simulink model "RBDmodel"  (R2023a)
settings: Solver=ode15s  StartTime=0.0  StopTime=4  FixedStep=0.0001  RelTol=1e-3  AbsTol=1e-3  EnableMultiTasking=on
model workspace (MAT data in the model file):
  C_Gimbal = 0.5
  C_IAP = 0.01
  IAP_Pa = 0
  K_Gimbal = 0
  K_IAP = 200
  LeftAbdominalMuscleForce = 0
  LeftBackMuscleForce = 0
  LeftTransverse1MuscleForce = 0
  LeftTransverse2MuscleForce = 0
  Moment_AR = 0
  Moment_FE = 7.5
  Moment_LB = 0
  RightAbdominalMuscleForce = 0
  RightBackMuscleForce = 0
  RightTransverse1MuscleForce = 0
  RightTransverse2MuscleForce = 0
  a = 1
  b = 1
  muscle_color = [0 0 1]
  muscle_radius = 1
libraries: checkpacklib x3, simulink x1
(part 1 of 2)
settings Model: PacingRate=0.110000  Creator=Siril TD  LastModifiedBy=siril
settings SolverCC: ZeroCrossAlgorithm=Adaptive  AutoInsertRateTranBlk=on
settings DataIOCC: LimitDataPoints=on  MaxDataPoints=50000  ReturnWorkspaceOutputsName=SDOSimTest_Log
settings OptimizationCC: LifeSpan=inf
settings DebuggingCC: IgnoredZcDiagnostic=none  UnconnectedInputMsg=warning  UnconnectedOutputMsg=warning  UnconnectedLineMsg=warning  AllowSymbolicDim=off  SFUnexpectedBacktrackingDiag=warning  SFNoUnconditionalDefaultTransitionDiag=warning  SFExecutionAtInitializationDiag=none  ArithmeticOperatorsInVariantConditions=warning
settings ModelReferenceCC: EnableRefExpFcnMdlSchedulingChecks=on
settings SFSimCC: SimUseLocalCustomCode=off  CustomCodeUndefinedFunction=UseInterfaceOnly
settings RTWCC: RTWUseLocalCustomCode=off  DLArmComputeVersion=19.05
settings CodeAppCC: StateflowObjectComments=on
settings GRTTargetCC: TargetLangStandard=C89/C90 (ANSI)
settings ConfigComp: CovMetricSettings=dw  CovSaveCumulativeToWorkspaceVar=on  CovSaveSingleToWorkspaceVar=on  CovExternalEMLEnable=off  CovSFcnEnable=off
settings SimscapeCC: SimscapeLogType=all  SimscapeLogSimulationStatistics=on  SimscapeLogDataHistory=10000

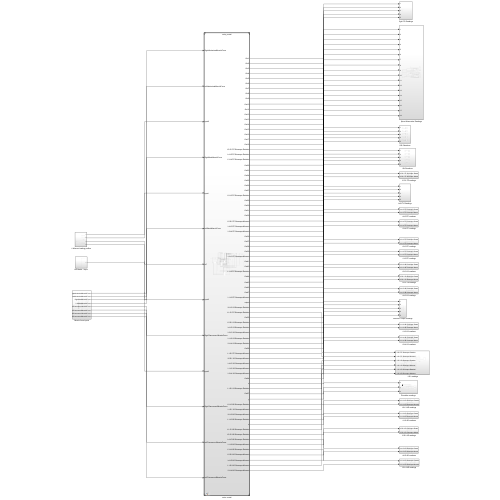
[thumbnail: Simulink's stored preview of the top-level diagram]
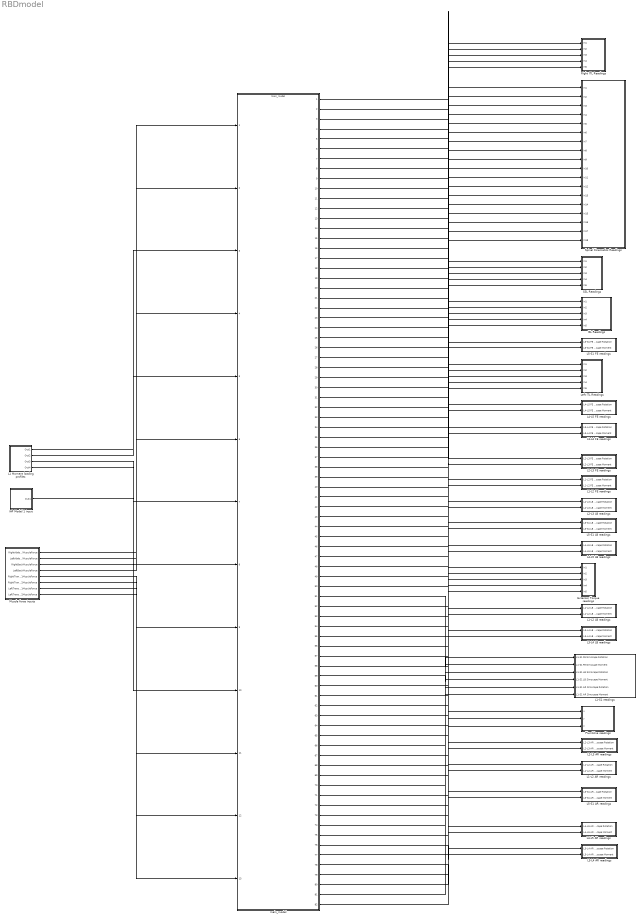
== system RBDmodel ==
  Extensor Torque readings : Subsystem
  IAP Model 1 input : Subsystem
  ISL Readings : Subsystem
  L1 Moment loading profiles : Subsystem
  L1-L2 AR readings : Subsystem
  L1-L2 FE readings : Subsystem
  L1-L2 LB readings : Subsystem
  L1-S1 readings : Subsystem
  L2-L3 AR readings : Subsystem
  L2-L3 FE readings : Subsystem
  L2-L3 LB readings : Subsystem
  L3-L4 AR readings : Subsystem
  L3-L4 FE readings : Subsystem
  L3-L4 LB readings : Subsystem
  L4-L5 AR readings : Subsystem
  L4-L5 FE readings : Subsystem
  L4-L5 LB readings : Subsystem
  L5-S1 AR readings : Subsystem
  L5-S1 FE readings : Subsystem
  L5-S1 LB readings : Subsystem
  Left ITL Readings : Subsystem
  Muscle force inputs : Subsystem
  Plumbline readings : Subsystem
  Right ITL Readings : Subsystem
  SSL Readings : Subsystem
  Spinal Kinematics Readings : Subsystem
  main_model : ModelReference  ModelNameDialog=main_model  SimulationMode=Normal  ModelReferenceVersion=6.155
  wires:
  main_model/20 -> L4-L5 FE readings/1(L4-L5 FE Simscape Rotation)
  main_model/67 -> Extensor Torque readings/5(In5)
  Muscle force inputs/4(LeftBackMuscleForce) -> main_model/6
  Muscle force inputs/3(RightBackMuscleForce) -> main_model/4
  L1 Moment loading profiles/1(Out1) -> main_model/3
  main_model/31 -> SSL Readings/4(In4)
  main_model/81 -> L1-S1 readings/6(L1-S1 AR Simscape Moment)
  main_model/56 -> L1-L2 LB readings/1(L1-L2 LB Simscape Rotation)
  L1 Moment loading profiles/2(Out2) -> main_model/5
  L1 Moment loading profiles/3(Out3) -> main_model/8
  main_model/50 -> L2-L3 LB readings/1(L2-L3 LB Simscape Rotation)
  main_model/6 -> SSL Readings/1(In1)
  L1 Moment loading profiles/4(Out4) -> main_model/10
  Muscle force inputs/1(RightAbdominalMuscleForce) -> main_model/1
  main_model/16 -> Left ITL Readings/2(In2)
  IAP Model 1 input/1(Out1) -> main_model/7
  Muscle force inputs/2(LeftAbdominalMuscleForce) -> main_model/2
  Muscle force inputs/5(RightTransverse1MuscleForce) -> main_model/9
  Muscle force inputs/6(RightTransverse2MuscleForce) -> main_model/11
  main_model/62 -> L1-L2 LB readings/2(L1-L2 LB Simscape Moment)
  Muscle force inputs/8(LeftTransverse2MuscleForce) -> main_model/13
  Muscle force inputs/7(LeftTransverse1MuscleForce) -> main_model/12
  main_model/63 -> L3-L4 LB readings/2(L3-L4 LB Simscape Moment)
  main_model/1 -> Spinal Kinematics Readings/1(In1)
  main_model/30 -> Spinal Kinematics Readings/13(In13)
  main_model/2 -> Spinal Kinematics Readings/2(In2)
  main_model/13 -> SSL Readings/2(In2)
  main_model/21 -> L3-L4 FE readings/1(L3-L4 FE Simscape Rotation)
  main_model/3 -> ISL Readings/1(In1)
  main_model/44 -> Spinal Kinematics Readings/17(In17)
  main_model/25 -> Spinal Kinematics Readings/11(In11)
  main_model/79 -> L5-S1 AR readings/2(L5-S1 AR Simscape Moment)
  main_model/4 -> Spinal Kinematics Readings/3(In3)
  main_model/5 -> Spinal Kinematics Readings/4(In4)
  main_model/77 -> L1-L2 AR readings/2(L1-L2 AR Simscape Moment)
  main_model/36 -> Spinal Kinematics Readings/14(In14)
  main_model/78 -> L3-L4 AR readings/1(L3-L4 AR Simscape Rotation)
  main_model/26 -> Left ITL Readings/3(In3)
  main_model/7 -> Spinal Kinematics Readings/5(In5)
  main_model/18 -> Right ITL Readings/3(In3)
  main_model/8 -> Left ITL Readings/1(In1)
  main_model/9 -> Right ITL Readings/1(In1)
  main_model/10 -> Spinal Kinematics Readings/6(In6)
  main_model/11 -> ISL Readings/2(In2)
  main_model/12 -> Spinal Kinematics Readings/7(In7)
  main_model/38 -> Left ITL Readings/4(In4)
  main_model/14 -> Right ITL Readings/2(In2)
  main_model/15 -> Spinal Kinematics Readings/8(In8)
  main_model/17 -> Spinal Kinematics Readings/9(In9)
  main_model/27 -> Right ITL Readings/4(In4)
  main_model/19 -> L5-S1 FE readings/1(L5-S1 FE Simscape Rotation)
  main_model/22 -> Spinal Kinematics Readings/10(In10)
  main_model/33 -> L5-S1 FE readings/2(L5-S1 FE Simscape Moment)
  main_model/23 -> ISL Readings/3(In3)
  main_model/45 -> Left ITL Readings/5(In5)
  main_model/24 -> SSL Readings/3(In3)
  main_model/28 -> L2-L3 FE readings/1(L2-L3 FE Simscape Rotation)
  main_model/29 -> Spinal Kinematics Readings/12(In12)
  main_model/32 -> Right ITL Readings/5(In5)
  main_model/34 -> L4-L5 FE readings/2(L4-L5 FE Simscape Moment)
  main_model/59 -> L1-S1 readings/2(L1-S1 FE Simscape Moment)
  main_model/35 -> L3-L4 FE readings/2(L3-L4 FE Simscape Moment)
  main_model/37 -> ISL Readings/4(In4)
  main_model/51 -> L1-S1 readings/1(L1-S1 FE Simscape Rotation)
  main_model/39 -> Spinal Kinematics Readings/15(In15)
  main_model/40 -> L2-L3 FE readings/2(L2-L3 FE Simscape Moment)
  main_model/41 -> Spinal Kinematics Readings/16(In16)
  main_model/42 -> SSL Readings/5(In5)
  main_model/43 -> L1-L2 FE readings/1(L1-L2 FE Simscape Rotation)
  main_model/46 -> Spinal Kinematics Readings/18(In18)
  main_model/47 -> ISL Readings/5(In5)
  main_model/48 -> L1-L2 FE readings/2(L1-L2 FE Simscape Moment)
  main_model/49 -> Extensor Torque readings/1(In1)
  main_model/52 -> Extensor Torque readings/2(In2)
  main_model/68 -> Plumbline readings/2(y)
  main_model/53 -> L5-S1 LB readings/1(L5-S1 LB Simscape Rotation)
  main_model/54 -> L4-L5 LB readings/1(L4-L5 LB Simscape Rotation)
  main_model/55 -> L2-L3 LB readings/2(L2-L3 LB Simscape Moment)
  main_model/57 -> L3-L4 LB readings/1(L3-L4 LB Simscape Rotation)
  main_model/58 -> Extensor Torque readings/3(In3)
  main_model/60 -> L5-S1 LB readings/2(L5-S1 LB Simscape Moment)
  main_model/61 -> L4-L5 LB readings/2(L4-L5 LB Simscape Moment)
  main_model/64 -> Extensor Torque readings/4(In4)
  main_model/65 -> Plumbline readings/1(x)
  main_model/66 -> L1-S1 readings/3(L1-S1 LB Simscape Rotation)
  main_model/69 -> L2-L3 AR readings/1(L2-L3 AR Simscape Rotation)
  main_model/70 -> L1-S1 readings/4(L1-S1 LB Simscape Moment)
  main_model/71 -> L2-L3 AR readings/2(L2-L3 AR Simscape Moment)
  main_model/72 -> L1-L2 AR readings/1(L1-L2 AR Simscape Rotation)
  main_model/73 -> Plumbline readings/3(z)
  main_model/74 -> L1-S1 readings/5(L1-S1 AR Simscape Rotation)
  main_model/75 -> L5-S1 AR readings/1(L5-S1 AR Simscape Rotation)
  main_model/76 -> L4-L5 AR readings/1(L4-L5 AR Simscape Rotation)
  main_model/80 -> L4-L5 AR readings/2(L4-L5 AR Simscape Moment)
  main_model/82 -> L3-L4 AR readings/2(L3-L4 AR Simscape Moment)

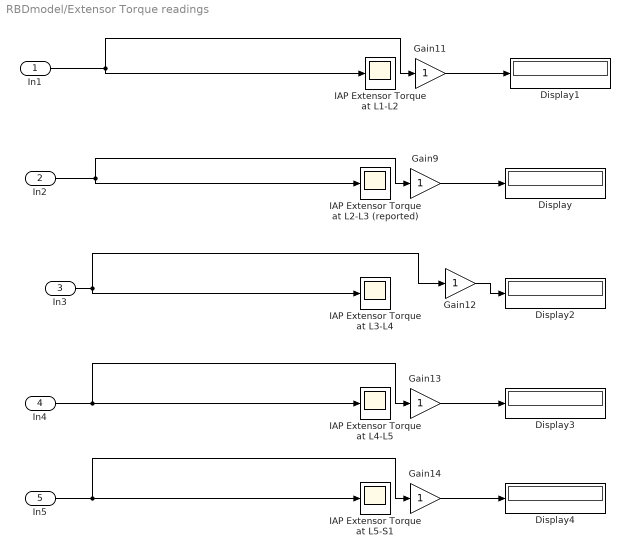
== system RBDmodel/Extensor Torque readings ==
  In1 : Inport
  In2 : Inport  Port=2
  In3 : Inport  Port=3
  In4 : Inport  Port=4
  In5 : Inport  Port=5
  Display{,1..4} (5 alike) : Display
      settings: Decimation=2
  Gain{9,11..14} (5 alike) : Gain
  IAP Extensor Torque at L1-L2 : Scope
  IAP Extensor Torque at L2-L3 (reported) : Scope
  IAP Extensor Torque at L3-L4 : Scope
  IAP Extensor Torque at L4-L5 : Scope
  IAP Extensor Torque at L5-S1 : Scope
  wires:
  Gain11/1 -> Display1/1
  Gain9/1 -> Display/1
  In5/1 -> Gain14/1, IAP Extensor Torque at L5-S1/1
  In2/1 -> Gain9/1, IAP Extensor Torque at L2-L3 (reported)/1
  Gain12/1 -> Display2/1
  In4/1 -> Gain13/1, IAP Extensor Torque at L4-L5/1
  In3/1 -> Gain12/1, IAP Extensor Torque at L3-L4/1
  Gain13/1 -> Display3/1
  In1/1 -> Gain11/1, IAP Extensor Torque at L1-L2/1
  Gain14/1 -> Display4/1

== system RBDmodel/IAP Model 1 input ==
  Constant96 : Constant  Value=IAP_Pa
  Out1 : Outport
  wires:
  Constant96/1 -> Out1/1

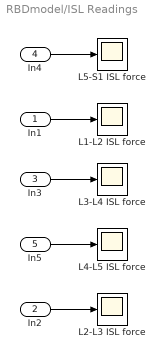
== system RBDmodel/ISL Readings ==
  In1 : Inport
  In2 : Inport  Port=2
  In3 : Inport  Port=3
  In4 : Inport  Port=4
  In5 : Inport  Port=5
  L1-L2 ISL force : Scope
  L2-L3 ISL force : Scope
  L3-L4 ISL force : Scope
  L4-L5 ISL force : Scope
  L5-S1 ISL force : Scope
  wires:
  In4/1 -> L5-S1 ISL force/1
  In2/1 -> L2-L3 ISL force/1
  In1/1 -> L1-L2 ISL force/1
  In3/1 -> L3-L4 ISL force/1
  In5/1 -> L4-L5 ISL force/1

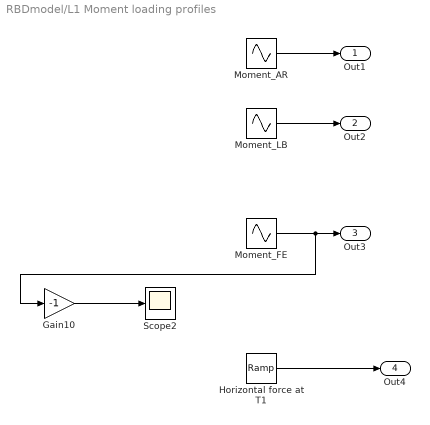
== system RBDmodel/L1 Moment loading profiles ==
  Gain10 : Gain  Gain=-1
  Horizontal force at T1 : simulink/Sources/Ramp  slope=0  start=0  InitialOutput=0
  Moment_AR : Sin  Amplitude=Moment_AR  SampleTime=0
  Moment_FE : Sin  Amplitude=-Moment_FE  SampleTime=0
  Moment_LB : Sin  Amplitude=-Moment_LB  SampleTime=0
  Scope2 : Scope
  Out1 : Outport
  Out2 : Outport  Port=2
  Out3 : Outport  Port=3
  Out4 : Outport  Port=4
  wires:
  Gain10/1 -> Scope2/1
  Horizontal force at T1/1 -> Out4/1
  Moment_LB/1 -> Out2/1
  Moment_AR/1 -> Out1/1
  Moment_FE/1 -> Gain10/1, Out3/1

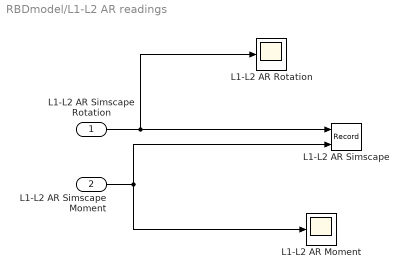
== system RBDmodel/L1-L2 AR readings ==
  L1-L2 AR Simscape Rotation : Inport
  L1-L2 AR Simscape Moment : Inport  Port=2
  L1-L2 AR Moment : Scope
  L1-L2 AR Rotation : Scope
  L1-L2 AR Simscape : Record  FileSettingsInternal="{\"entries\":[{\"content\":{\"excelSettings\":{\"content\":{},\"type\":\"Streamout.ExcelSettings\"}},\"type\":\"Streamout.FileSettingStorage\",\"uuid\":\"b28dc066-991e-4613-a00d-d29ff6d798a1\"}],\"packageUris\":[\"http://schema.mathworks.com/mf0/streamout_blocks/R2020a\"],\"version\":\"1.0\"}"  Layout=[1 1]  SignalsInternal="{\"entries\":[{\"content\":{\"signals\":[{\"content\":{\"blockPath\":[\"RBDmodel/L1-L2 AR readings/L1-L2 AR Simscape\"],\"dimensions\":[1],\"domain\":\"RBDmodel/L1-L2 AR readings/L1-L2 AR Simscape\",\"lineColor\":\"#ff6929\",\"port\":1,\"sid\":[\"\"],\"signalID\":1360,\"signalName\":\"L1-L2 AR Simscape Rotation\"},\"type\":\"RecordBlkView.Signal\",\"uuid\":\"012eb32e-fa43-42f2-9214-58300afc2241\"},{\"content\":{\"blockPath\":[\"RBDmodel/L1-L2 AR readings/L1-L2 AR Simscape\"],\"dimensions\":[1],\"domain\":\"RBDmodel/L1-L2 AR readings/L1-L2 AR Simscape\",\"lineColor\":\"#b746ff\",\"port\":2,\"sid\":[\"\"],\"signalID\":1364,\"signalName\":\"L1-L2 AR Simscape Moment\"},\"type\":\"RecordBlkView.Signal\",\"uuid\":\"1a3da7e1-f63f-4174-9c92-f6b8960343b7\"}]},\"type\":\"RecordBlkView.InputSignals\",\"uuid\":\"afe20b8d-c1d7-4091-a686-51fac02b3391\"}],\"packageUris\":[\"http://schema.mathworks.com/mf0/streamout_blocks/R2020a\"],\"version\":\"1.0\"}"  VisualizationBindings="{\"xyplotplugin\":{\"info\":[{\"series\":[],\"subplotID\":1}]}}"  CompatibilityTag=XY
  wires:
  L1-L2 AR Simscape Rotation/1 -> L1-L2 AR Simscape/1, L1-L2 AR Rotation/1
  L1-L2 AR Simscape Moment/1 -> L1-L2 AR Simscape/2, L1-L2 AR Moment/1

== system RBDmodel/L1-L2 FE readings ==
  L1-L2 FE Simscape Rotation : Inport
  L1-L2 FE Simscape Moment : Inport  Port=2
  L1-L2 FE Moment : Scope
  L1-L2 FE Rotation : Scope
  L1-L2 FE Simscape : Record  FileSettingsInternal="{\"entries\":[{\"content\":{\"excelSettings\":{\"content\":{},\"type\":\"Streamout.ExcelSettings\"}},\"type\":\"Streamout.FileSettingStorage\",\"uuid\":\"8ce7ea1e-727d-4085-a2f9-c3a4a6f5bb0a\"}],\"packageUris\":[\"http://schema.mathworks.com/mf0/streamout_blocks/R2020a\"],\"version\":\"1.0\"}"  Layout=[1 1]  SignalsInternal="{\"entries\":[{\"content\":{\"signals\":[{\"content\":{\"blockPath\":[\"RBDmodel/L1-L2 FE readings/L1-L2 FE Simscape\"],\"dimensions\":[1],\"domain\":\"RBDmodel/L1-L2 FE readings/L1-L2 FE Simscape\",\"lineColor\":\"#64d413\",\"port\":1,\"sid\":[\"\"],\"signalID\":1368,\"signalName\":\"L1-L2 FE Simscape Rotation\"},\"type\":\"RecordBlkView.Signal\",\"uuid\":\"14272d5e-dfd7-46c4-858f-28ca2b9ba15c\"},{\"content\":{\"blockPath\":[\"RBDmodel/L1-L2 FE readings/L1-L2 FE Simscape\"],\"dimensions\":[1],\"domain\":\"RBDmodel/L1-L2 FE readings/L1-L2 FE Simscape\",\"lineColor\":\"#ff13a6\",\"port\":2,\"sid\":[\"\"],\"signalID\":1372,\"signalName\":\"L1-L2 FE Simscape Moment\"},\"type\":\"RecordBlkView.Signal\",\"uuid\":\"e4bc809e-e80f-4428-925d-a05f0499dadb\"}]},\"type\":\"RecordBlkView.InputSignals\",\"uuid\":\"2abea1ec-8224-445c-bef5-2230a40efcc7\"}],\"packageUris\":[\"http://schema.mathworks.com/mf0/streamout_blocks/R2020a\"],\"version\":\"1.0\"}"  VisualizationBindings="{\"xyplotplugin\":{\"info\":[{\"series\":[],\"subplotID\":1}]}}"  CompatibilityTag=XY
  wires:
  L1-L2 FE Simscape Rotation/1 -> L1-L2 FE Simscape/1, L1-L2 FE Rotation/1
  L1-L2 FE Simscape Moment/1 -> L1-L2 FE Simscape/2, L1-L2 FE Moment/1

== system RBDmodel/L1-L2 LB readings ==
  L1-L2 LB Simscape Rotation : Inport
  L1-L2 LB Simscape Moment : Inport  Port=2
  L1-L2 LB Moment : Scope
  L1-L2 LB Rotation : Scope
  L1-L2 LB Simscape : Record  FileSettingsInternal="{\"entries\":[{\"content\":{\"excelSettings\":{\"content\":{},\"type\":\"Streamout.ExcelSettings\"}},\"type\":\"Streamout.FileSettingStorage\",\"uuid\":\"f91b6da8-1a5e-44a2-9c0b-2edd10b764e6\"}],\"packageUris\":[\"http://schema.mathworks.com/mf0/streamout_blocks/R2020a\"],\"version\":\"1.0\"}"  Layout=[1 1]  SignalsInternal="{\"entries\":[{\"content\":{\"signals\":[{\"content\":{\"blockPath\":[\"RBDmodel/L1-L2 LB readings/L1-L2 LB Simscape\"],\"dimensions\":[1],\"domain\":\"RBDmodel/L1-L2 LB readings/L1-L2 LB Simscape\",\"lineColor\":\"#fe330a\",\"port\":1,\"sid\":[\"\"],\"signalID\":1376,\"signalName\":\"L1-L2 LB Simscape Rotation\"},\"type\":\"RecordBlkView.Signal\",\"uuid\":\"621c9457-627a-42f5-82bc-3f73ddf07535\"},{\"content\":{\"blockPath\":[\"RBDmodel/L1-L2 LB readings/L1-L2 LB Simscape\"],\"dimensions\":[1],\"domain\":\"RBDmodel/L1-L2 LB readings/L1-L2 LB Simscape\",\"lineColor\":\"#22b573\",\"port\":2,\"sid\":[\"\"],\"signalID\":1380,\"signalName\":\"L1-L2 LB Simscape Moment\"},\"type\":\"RecordBlkView.Signal\",\"uuid\":\"2edc97f2-ad54-4451-8d37-6e34baaded79\"}]},\"type\":\"RecordBlkView.InputSignals\",\"uuid\":\"6599f76d-7cc0-48aa-b01b-dd0004c97a2e\"}],\"packageUris\":[\"http://schema.mathworks.com/mf0/streamout_blocks/R2020a\"],\"version\":\"1.0\"}"  VisualizationBindings="{\"xyplotplugin\":{\"info\":[{\"series\":[],\"subplotID\":1}]}}"  CompatibilityTag=XY
  wires:
  L1-L2 LB Simscape Moment/1 -> L1-L2 LB Simscape/2, L1-L2 LB Moment/1
  L1-L2 LB Simscape Rotation/1 -> L1-L2 LB Simscape/1, L1-L2 LB Rotation/1

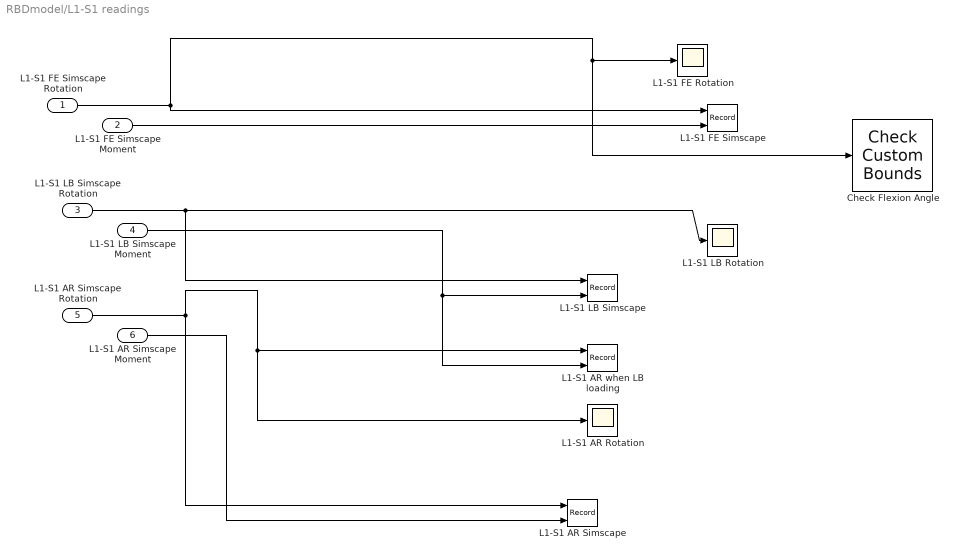
== system RBDmodel/L1-S1 readings ==
  L1-S1 FE Simscape Rotation : Inport
  L1-S1 FE Simscape Moment : Inport  Port=2
  L1-S1 LB Simscape Rotation : Inport  Port=3
  L1-S1 LB Simscape Moment : Inport  Port=4
  L1-S1 AR Simscape Rotation : Inport  Port=5
  L1-S1 AR Simscape Moment : Inport  Port=6
  Check Flexion Angle : checkpacklib/Check Custom Bounds  InstantiateOnLoad=on  enabled=off  stopWhenAssertionFail=off  export=off  ViewDlgPos=[100 200 510 390]  OpenViewOnLoad=off  LaunchViewOnOpen=off  TimeUnits=seconds  EnableUpperBound=on  UpperBoundTimes=[5 10]  UpperBoundAmplitudes=[51 51];  EnableLowerBound=on  LowerBoundTimes=[6 10]  LowerBoundAmplitudes=[49 49];
      settings: LibrarySourceBlock=sdolib/Signal Constraints/Check Custom Bounds
  L1-S1 AR Rotation : Scope
  L1-S1 AR Simscape : Record  FileSettingsInternal="{\"entries\":[{\"content\":{\"excelSettings\":{\"content\":{},\"type\":\"Streamout.ExcelSettings\"}},\"type\":\"Streamout.FileSettingStorage\",\"uuid\":\"b954e3b6-b992-4288-8e9e-83c0e0eed84f\"}],\"packageUris\":[\"http://schema.mathworks.com/mf0/streamout_blocks/R2020a\"],\"version\":\"1.0\"}"  Layout=[1 1]  SignalsInternal="{\"entries\":[{\"content\":{\"signals\":[{\"content\":{\"blockPath\":[\"RBDmodel/L1-S1 readings/L1-S1 AR Simscape\"],\"dimensions\":[1,1],\"domain\":\"RBDmodel/L1-S1 readings/L1-S1 AR Simscape\",\"lineColor\":\"#edb120\",\"port\":1,\"sid\":[\"\"],\"signalID\":1392,\"signalName\":\"L1-S1 AR Simscape Rotation\"},\"type\":\"RecordBlkView.Signal\",\"uuid\":\"797d9295-84dd-4e98-b2bd-abb01ffb65f1\"},{\"content\":{\"blockPath\":[\"RBDmodel/L1-S1 readings/L1-S1 AR Simscape\"],\"dimensions\":[1],\"domain\":\"RBDmodel/L1-S1 readings/L1-S1 AR Simscape\",\"lineColor\":\"#7e2f8e\",\"port\":2,\"sid\":[\"\"],\"signalID\":1396,\"signalName\":\"L1-S1 AR Simscape Moment\"},\"type\":\"RecordBlkView.Signal\",\"uuid\":\"1e31dda2-2ea6-4a38-a0e0-59a33a30f3aa\"}]},\"type\":\"RecordBlkView.InputSignals\",\"uuid\":\"77442a82-e315-402b-8b1a-300b9592f177\"}],\"packageUris\":[\"http://schema.mathworks.com/mf0/streamout_blocks/R2020a\"],\"version\":\"1.0\"}"  VisualizationBindings="{\"xyplotplugin\":{\"info\":[{\"series\":[],\"subplotID\":1}]}}"  CompatibilityTag=XY
  L1-S1 AR when LB loading : Record  FileSettingsInternal="{\"entries\":[{\"content\":{\"excelSettings\":{\"content\":{},\"type\":\"Streamout.ExcelSettings\"}},\"type\":\"Streamout.FileSettingStorage\",\"uuid\":\"7c9a55b9-26e2-4dee-8ab6-75e3d662341a\"}],\"packageUris\":[\"http://schema.mathworks.com/mf0/streamout_blocks/R2020a\"],\"version\":\"1.0\"}"  Layout=[1 1]  SignalsInternal="{\"entries\":[{\"content\":{\"signals\":[{\"content\":{\"blockPath\":[\"RBDmodel/L1-S1 readings/L1-S1 AR when LB loading\"],\"dimensions\":[1,1],\"domain\":\"RBDmodel/L1-S1 readings/L1-S1 AR when LB loading\",\"lineColor\":\"#77ac30\",\"port\":1,\"sid\":[\"\"],\"signalID\":1400,\"signalName\":\"L1-S1 AR Simscape Rotation\"},\"type\":\"RecordBlkView.Signal\",\"uuid\":\"fc9ea2b7-01a5-4fec-8c12-8ed0258352bf\"},{\"content\":{\"blockPath\":[\"RBDmodel/L1-S1 readings/L1-S1 AR when LB loading\"],\"dimensions\":[1],\"domain\":\"RBDmodel/L1-S1 readings/L1-S1 AR when LB loading\",\"lineColor\":\"#4dbeee\",\"port\":2,\"sid\":[\"\"],\"signalID\":1404,\"signalName\":\"L1-S1 LB Simscape Moment\"},\"type\":\"RecordBlkView.Signal\",\"uuid\":\"99554ea6-9241-406f-a7ff-00c072a0b4e4\"}]},\"type\":\"RecordBlkView.InputSignals\",\"uuid\":\"3f4efdd9-c46f-425d-a98a-f481f6a35fee\"}],\"packageUris\":[\"http://schema.mathworks.com/mf0/streamout_blocks/R2020a\"],\"version\":\"1.0\"}"  VisualizationBindings="{\"xyplotplugin\":{\"info\":[{\"series\":[],\"subplotID\":1}]}}"  CompatibilityTag=XY
  L1-S1 FE Rotation : Scope
  L1-S1 FE Simscape : Record  FileSettingsInternal="{\"entries\":[{\"content\":{\"excelSettings\":{\"content\":{},\"type\":\"Streamout.ExcelSettings\"}},\"type\":\"Streamout.FileSettingStorage\",\"uuid\":\"4277ec63-d6bc-434d-a603-e60f5b770cfc\"}],\"packageUris\":[\"http://schema.mathworks.com/mf0/streamout_blocks/R2020a\"],\"version\":\"1.0\"}"  Layout=[1 1]  SignalsInternal="{\"entries\":[{\"content\":{\"signals\":[{\"content\":{\"blockPath\":[\"RBDmodel/L1-S1 readings/L1-S1 FE Simscape\"],\"dimensions\":[1,1],\"domain\":\"RBDmodel/L1-S1 readings/L1-S1 FE Simscape\",\"lineColor\":\"#0072bd\",\"port\":1,\"sid\":[\"\"],\"signalID\":1384,\"signalName\":\"L1-S1 FE Simscape Rotation\"},\"type\":\"RecordBlkView.Signal\",\"uuid\":\"b05b0e40-1441-4de0-b556-a25aa3c4cf09\"},{\"content\":{\"blockPath\":[\"RBDmodel/L1-S1 readings/L1-S1 FE Simscape\"],\"dimensions\":[1],\"domain\":\"RBDmodel/L1-S1 readings/L1-S1 FE Simscape\",\"lineColor\":\"#d95319\",\"port\":2,\"sid\":[\"\"],\"signalID\":1388,\"signalName\":\"L1-S1 FE Simscape Moment\"},\"type\":\"RecordBlkView.Signal\",\"uuid\":\"32cda3f8-6cbe-4181-ae22-8066d64c7fad\"}]},\"type\":\"RecordBlkView.InputSignals\",\"uuid\":\"42077291-aac0-4e4f-98f6-8f120505d114\"}],\"packageUris\":[\"http://schema.mathworks.com/mf0/streamout_blocks/R2020a\"],\"version\":\"1.0\"}"  VisualizationBindings="{\"xyplotplugin\":{\"info\":[{\"series\":[],\"subplotID\":1}]}}"  CompatibilityTag=XY
  L1-S1 LB Rotation : Scope
  L1-S1 LB Simscape : Record  FileSettingsInternal="{\"entries\":[{\"content\":{\"excelSettings\":{\"content\":{},\"type\":\"Streamout.ExcelSettings\"}},\"type\":\"Streamout.FileSettingStorage\",\"uuid\":\"d051a5cc-fb2e-466c-bd05-561f4ba50a96\"}],\"packageUris\":[\"http://schema.mathworks.com/mf0/streamout_blocks/R2020a\"],\"version\":\"1.0\"}"  Layout=[1 1]  SignalsInternal="{\"entries\":[{\"content\":{\"signals\":[{\"content\":{\"blockPath\":[\"RBDmodel/L1-S1 readings/L1-S1 LB Simscape\"],\"dimensions\":[1,1],\"domain\":\"RBDmodel/L1-S1 readings/L1-S1 LB Simscape\",\"lineColor\":\"#a2142f\",\"port\":1,\"sid\":[\"\"],\"signalID\":1408,\"signalName\":\"L1-S1 LB Simscape Rotation\"},\"type\":\"RecordBlkView.Signal\",\"uuid\":\"a043fbb2-f081-461b-bfbf-22b79d9b12f8\"},{\"content\":{\"blockPath\":[\"RBDmodel/L1-S1 readings/L1-S1 LB Simscape\"],\"dimensions\":[1],\"domain\":\"RBDmodel/L1-S1 readings/L1-S1 LB Simscape\",\"lineColor\":\"#139fff\",\"port\":2,\"sid\":[\"\"],\"signalID\":1412,\"signalName\":\"L1-S1 LB Simscape Moment\"},\"type\":\"RecordBlkView.Signal\",\"uuid\":\"92bbd904-5685-4112-b61d-6e93200ea034\"}]},\"type\":\"RecordBlkView.InputSignals\",\"uuid\":\"6b8d1cb8-5b8d-4fed-9469-309b6002e987\"}],\"packageUris\":[\"http://schema.mathworks.com/mf0/streamout_blocks/R2020a\"],\"version\":\"1.0\"}"  VisualizationBindings="{\"xyplotplugin\":{\"info\":[{\"series\":[],\"subplotID\":1}]}}"  CompatibilityTag=XY
  wires:
  L1-S1 LB Simscape Rotation/1 -> L1-S1 LB Simscape/1, L1-S1 LB Rotation/1
  L1-S1 FE Simscape Rotation/1 -> Check Flexion Angle/1, L1-S1 FE Rotation/1, L1-S1 FE Simscape/1
  L1-S1 AR Simscape Rotation/1 -> L1-S1 AR when LB loading/1, L1-S1 AR Rotation/1, L1-S1 AR Simscape/1
  L1-S1 LB Simscape Moment/1 -> L1-S1 LB Simscape/2, L1-S1 AR when LB loading/2
  L1-S1 FE Simscape Moment/1 -> L1-S1 FE Simscape/2
  L1-S1 AR Simscape Moment/1 -> L1-S1 AR Simscape/2

== system RBDmodel/L2-L3 AR readings ==
  L2-L3 AR Simscape Rotation : Inport
  L2-L3 AR Simscape Moment : Inport  Port=2
  L2-L3 AR Moment : Scope
  L2-L3 AR Rotation : Scope
  L2-L3 AR Simscape : Record  FileSettingsInternal="{\"entries\":[{\"content\":{\"excelSettings\":{\"content\":{},\"type\":\"Streamout.ExcelSettings\"}},\"type\":\"Streamout.FileSettingStorage\",\"uuid\":\"1b3dca45-e25d-4c43-83f1-4bff6aa87f96\"}],\"packageUris\":[\"http://schema.mathworks.com/mf0/streamout_blocks/R2020a\"],\"version\":\"1.0\"}"  Layout=[1 1]  SignalsInternal="{\"entries\":[{\"content\":{\"signals\":[{\"content\":{\"blockPath\":[\"RBDmodel/L2-L3 AR readings/L2-L3 AR Simscape\"],\"dimensions\":[1],\"domain\":\"RBDmodel/L2-L3 AR readings/L2-L3 AR Simscape\",\"lineColor\":\"#ff6929\",\"port\":1,\"sid\":[\"\"],\"signalID\":1416,\"signalName\":\"L2-L3 AR Simscape Rotation\"},\"type\":\"RecordBlkView.Signal\",\"uuid\":\"e70d2628-5331-497c-85aa-337cd48ba713\"},{\"content\":{\"blockPath\":[\"RBDmodel/L2-L3 AR readings/L2-L3 AR Simscape\"],\"dimensions\":[1],\"domain\":\"RBDmodel/L2-L3 AR readings/L2-L3 AR Simscape\",\"lineColor\":\"#b746ff\",\"port\":2,\"sid\":[\"\"],\"signalID\":1420,\"signalName\":\"L2-L3 AR Simscape Moment\"},\"type\":\"RecordBlkView.Signal\",\"uuid\":\"af39c3ea-201a-40c1-a483-dfe03c7ab99b\"}]},\"type\":\"RecordBlkView.InputSignals\",\"uuid\":\"a20d0424-911b-47f8-ba88-4e87d1c9c6ef\"}],\"packageUris\":[\"http://schema.mathworks.com/mf0/streamout_blocks/R2020a\"],\"version\":\"1.0\"}"  VisualizationBindings="{\"xyplotplugin\":{\"info\":[{\"series\":[],\"subplotID\":1}]}}"  CompatibilityTag=XY
  wires:
  L2-L3 AR Simscape Rotation/1 -> L2-L3 AR Simscape/1, L2-L3 AR Rotation/1
  L2-L3 AR Simscape Moment/1 -> L2-L3 AR Simscape/2, L2-L3 AR Moment/1

== system RBDmodel/L2-L3 FE readings ==
  L2-L3 FE Simscape Rotation : Inport
  L2-L3 FE Simscape Moment : Inport  Port=2
  L2-L3 FE Moment : Scope
  L2-L3 FE Rotation : Scope
  L2-L3 FE Simscape : Record  FileSettingsInternal="{\"entries\":[{\"content\":{\"excelSettings\":{\"content\":{},\"type\":\"Streamout.ExcelSettings\"}},\"type\":\"Streamout.FileSettingStorage\",\"uuid\":\"a8dbeb5b-ff1f-49c5-807a-ed83070a13e0\"}],\"packageUris\":[\"http://schema.mathworks.com/mf0/streamout_blocks/R2020a\"],\"version\":\"1.0\"}"  Layout=[1 1]  SignalsInternal="{\"entries\":[{\"content\":{\"signals\":[{\"content\":{\"blockPath\":[\"RBDmodel/L2-L3 FE readings/L2-L3 FE Simscape\"],\"dimensions\":[1],\"domain\":\"RBDmodel/L2-L3 FE readings/L2-L3 FE Simscape\",\"lineColor\":\"#64d413\",\"port\":1,\"sid\":[\"\"],\"signalID\":1424,\"signalName\":\"L2-L3 FE Simscape Rotation\"},\"type\":\"RecordBlkView.Signal\",\"uuid\":\"610a7a81-37ad-4730-b63c-a5761efec7a8\"},{\"content\":{\"blockPath\":[\"RBDmodel/L2-L3 FE readings/L2-L3 FE Simscape\"],\"dimensions\":[1],\"domain\":\"RBDmodel/L2-L3 FE readings/L2-L3 FE Simscape\",\"lineColor\":\"#ff13a6\",\"port\":2,\"sid\":[\"\"],\"signalID\":1428,\"signalName\":\"L2-L3 FE Simscape Moment\"},\"type\":\"RecordBlkView.Signal\",\"uuid\":\"85b15c0e-062c-4388-a88e-8c4ab91d18f2\"}]},\"type\":\"RecordBlkView.InputSignals\",\"uuid\":\"8aa61301-8cd2-4db8-affe-7794c216c0d9\"}],\"packageUris\":[\"http://schema.mathworks.com/mf0/streamout_blocks/R2020a\"],\"version\":\"1.0\"}"  VisualizationBindings="{\"xyplotplugin\":{\"info\":[{\"series\":[],\"subplotID\":1}]}}"  CompatibilityTag=XY
  wires:
  L2-L3 FE Simscape Rotation/1 -> L2-L3 FE Simscape/1, L2-L3 FE Rotation/1
  L2-L3 FE Simscape Moment/1 -> L2-L3 FE Simscape/2, L2-L3 FE Moment/1

== system RBDmodel/L2-L3 LB readings ==
  L2-L3 LB Simscape Rotation : Inport
  L2-L3 LB Simscape Moment : Inport  Port=2
  L2-L3 LB Moment : Scope
  L2-L3 LB Rotation : Scope
  L2-L3 LB Simscape : Record  FileSettingsInternal="{\"entries\":[{\"content\":{\"excelSettings\":{\"content\":{},\"type\":\"Streamout.ExcelSettings\"}},\"type\":\"Streamout.FileSettingStorage\",\"uuid\":\"ebb8c812-f4e5-4f1b-bb26-5cc9383d42b0\"}],\"packageUris\":[\"http://schema.mathworks.com/mf0/streamout_blocks/R2020a\"],\"version\":\"1.0\"}"  Layout=[1 1]  SignalsInternal="{\"entries\":[{\"content\":{\"signals\":[{\"content\":{\"blockPath\":[\"RBDmodel/L2-L3 LB readings/L2-L3 LB Simscape\"],\"dimensions\":[1],\"domain\":\"RBDmodel/L2-L3 LB readings/L2-L3 LB Simscape\",\"lineColor\":\"#fe330a\",\"port\":1,\"sid\":[\"\"],\"signalID\":1432,\"signalName\":\"L2-L3 LB Simscape Rotation\"},\"type\":\"RecordBlkView.Signal\",\"uuid\":\"54576e5c-c28b-43e4-9224-e94e1705c380\"},{\"content\":{\"blockPath\":[\"RBDmodel/L2-L3 LB readings/L2-L3 LB Simscape\"],\"dimensions\":[1],\"domain\":\"RBDmodel/L2-L3 LB readings/L2-L3 LB Simscape\",\"lineColor\":\"#22b573\",\"port\":2,\"sid\":[\"\"],\"signalID\":1436,\"signalName\":\"L2-L3 LB Simscape Moment\"},\"type\":\"RecordBlkView.Signal\",\"uuid\":\"a9740b53-4785-48f0-9501-c2b6069bd585\"}]},\"type\":\"RecordBlkView.InputSignals\",\"uuid\":\"1bea8120-5db7-433b-aae0-c9997d8e4541\"}],\"packageUris\":[\"http://schema.mathworks.com/mf0/streamout_blocks/R2020a\"],\"version\":\"1.0\"}"  VisualizationBindings="{\"xyplotplugin\":{\"info\":[{\"series\":[],\"subplotID\":1}]}}"  CompatibilityTag=XY
  wires:
  L2-L3 LB Simscape Rotation/1 -> L2-L3 LB Simscape/1, L2-L3 LB Rotation/1
  L2-L3 LB Simscape Moment/1 -> L2-L3 LB Simscape/2, L2-L3 LB Moment/1

== system RBDmodel/L3-L4 AR readings ==
  L3-L4 AR Simscape Rotation : Inport
  L3-L4 AR Simscape Moment : Inport  Port=2
  L3-L4 AR Moment : Scope
  L3-L4 AR Rotation : Scope
  L3-L4 AR Simscape : Record  FileSettingsInternal="{\"entries\":[{\"content\":{\"excelSettings\":{\"content\":{},\"type\":\"Streamout.ExcelSettings\"}},\"type\":\"Streamout.FileSettingStorage\",\"uuid\":\"0d852f55-8e65-459e-b217-a04e03d20f27\"}],\"packageUris\":[\"http://schema.mathworks.com/mf0/streamout_blocks/R2020a\"],\"version\":\"1.0\"}"  Layout=[1 1]  SignalsInternal="{\"entries\":[{\"content\":{\"signals\":[{\"content\":{\"blockPath\":[\"RBDmodel/L3-L4 AR readings/L3-L4 AR Simscape\"],\"dimensions\":[1],\"domain\":\"RBDmodel/L3-L4 AR readings/L3-L4 AR Simscape\",\"lineColor\":\"#0072bd\",\"port\":1,\"sid\":[\"\"],\"signalID\":1440,\"signalName\":\"L3-L4 AR Simscape Rotation\"},\"type\":\"RecordBlkView.Signal\",\"uuid\":\"751fb338-a416-415f-9a67-fed1a750ab96\"},{\"content\":{\"blockPath\":[\"RBDmodel/L3-L4 AR readings/L3-L4 AR Simscape\"],\"dimensions\":[1],\"domain\":\"RBDmodel/L3-L4 AR readings/L3-L4 AR Simscape\",\"lineColor\":\"#d95319\",\"port\":2,\"sid\":[\"\"],\"signalID\":1444,\"signalName\":\"L3-L4 AR Simscape Moment\"},\"type\":\"RecordBlkView.Signal\",\"uuid\":\"1623f842-dbcd-465f-acad-6502715e33f9\"}]},\"type\":\"RecordBlkView.InputSignals\",\"uuid\":\"4d0e25ad-78aa-47cf-9e32-c99cd5c12085\"}],\"packageUris\":[\"http://schema.mathworks.com/mf0/streamout_blocks/R2020a\"],\"version\":\"1.0\"}"  VisualizationBindings="{\"xyplotplugin\":{\"info\":[{\"series\":[],\"subplotID\":1}]}}"  CompatibilityTag=XY
  wires:
  L3-L4 AR Simscape Rotation/1 -> L3-L4 AR Simscape/1, L3-L4 AR Rotation/1
  L3-L4 AR Simscape Moment/1 -> L3-L4 AR Simscape/2, L3-L4 AR Moment/1

== system RBDmodel/L3-L4 FE readings ==
  L3-L4 FE Simscape Rotation : Inport
  L3-L4 FE Simscape Moment : Inport  Port=2
  L3-L4 FE Moment : Scope
  L3-L4 FE Rotation : Scope
  L3-L4 FE Simscape : Record  FileSettingsInternal="{\"entries\":[{\"content\":{\"excelSettings\":{\"content\":{},\"type\":\"Streamout.ExcelSettings\"}},\"type\":\"Streamout.FileSettingStorage\",\"uuid\":\"4a97007c-b2c5-4a2b-a22c-db91ba4f89a2\"}],\"packageUris\":[\"http://schema.mathworks.com/mf0/streamout_blocks/R2020a\"],\"version\":\"1.0\"}"  Layout=[1 1]  SignalsInternal="{\"entries\":[{\"content\":{\"signals\":[{\"content\":{\"blockPath\":[\"RBDmodel/L3-L4 FE readings/L3-L4 FE Simscape\"],\"dimensions\":[1],\"domain\":\"RBDmodel/L3-L4 FE readings/L3-L4 FE Simscape\",\"lineColor\":\"#edb120\",\"port\":1,\"sid\":[\"\"],\"signalID\":1448,\"signalName\":\"L3-L4 FE Simscape Rotation\"},\"type\":\"RecordBlkView.Signal\",\"uuid\":\"77a480f7-8074-47be-8fdf-a8caa3efc9ea\"},{\"content\":{\"blockPath\":[\"RBDmodel/L3-L4 FE readings/L3-L4 FE Simscape\"],\"dimensions\":[1],\"domain\":\"RBDmodel/L3-L4 FE readings/L3-L4 FE Simscape\",\"lineColor\":\"#7e2f8e\",\"port\":2,\"sid\":[\"\"],\"signalID\":1452,\"signalName\":\"L3-L4 FE Simscape Moment\"},\"type\":\"RecordBlkView.Signal\",\"uuid\":\"bbaedb1d-6b55-4b73-9374-f86fb5d1519f\"}]},\"type\":\"RecordBlkView.InputSignals\",\"uuid\":\"8922dd5c-60c6-4104-bd66-638812c4d691\"}],\"packageUris\":[\"http://schema.mathworks.com/mf0/streamout_blocks/R2020a\"],\"version\":\"1.0\"}"  VisualizationBindings="{\"xyplotplugin\":{\"info\":[{\"series\":[],\"subplotID\":1}]}}"  CompatibilityTag=XY
  wires:
  L3-L4 FE Simscape Rotation/1 -> L3-L4 FE Simscape/1, L3-L4 FE Rotation/1
  L3-L4 FE Simscape Moment/1 -> L3-L4 FE Simscape/2, L3-L4 FE Moment/1

== system RBDmodel/L3-L4 LB readings ==
  L3-L4 LB Simscape Rotation : Inport
  L3-L4 LB Simscape Moment : Inport  Port=2
  L3-L4 LB Moment : Scope
  L3-L4 LB Rotation : Scope
  L3-L4 LB Simscape : Record  FileSettingsInternal="{\"entries\":[{\"content\":{\"excelSettings\":{\"content\":{},\"type\":\"Streamout.ExcelSettings\"}},\"type\":\"Streamout.FileSettingStorage\",\"uuid\":\"1c058524-eb60-4b6f-8fef-1b5d5278ec82\"}],\"packageUris\":[\"http://schema.mathworks.com/mf0/streamout_blocks/R2020a\"],\"version\":\"1.0\"}"  Layout=[1 1]  SignalsInternal="{\"entries\":[{\"content\":{\"signals\":[{\"content\":{\"blockPath\":[\"RBDmodel/L3-L4 LB readings/L3-L4 LB Simscape\"],\"dimensions\":[1],\"domain\":\"RBDmodel/L3-L4 LB readings/L3-L4 LB Simscape\",\"lineColor\":\"#77ac30\",\"port\":1,\"sid\":[\"\"],\"signalID\":1456,\"signalName\":\"L3-L4 LB Simscape Rotation\"},\"type\":\"RecordBlkView.Signal\",\"uuid\":\"2dc6856a-0e52-4543-b3ac-6e8ed32a5d94\"},{\"content\":{\"blockPath\":[\"RBDmodel/L3-L4 LB readings/L3-L4 LB Simscape\"],\"dimensions\":[1],\"domain\":\"RBDmodel/L3-L4 LB readings/L3-L4 LB Simscape\",\"lineColor\":\"#4dbeee\",\"port\":2,\"sid\":[\"\"],\"signalID\":1460,\"signalName\":\"L3-L4 LB Simscape Moment\"},\"type\":\"RecordBlkView.Signal\",\"uuid\":\"eb138c01-ee40-4649-b1c0-29d03f62432c\"}]},\"type\":\"RecordBlkView.InputSignals\",\"uuid\":\"c7c7ce33-7e8f-4fb1-9a81-42256479e298\"}],\"packageUris\":[\"http://schema.mathworks.com/mf0/streamout_blocks/R2020a\"],\"version\":\"1.0\"}"  VisualizationBindings="{\"xyplotplugin\":{\"info\":[{\"series\":[],\"subplotID\":1}]}}"  CompatibilityTag=XY
  wires:
  L3-L4 LB Simscape Rotation/1 -> L3-L4 LB Simscape/1, L3-L4 LB Rotation/1
  L3-L4 LB Simscape Moment/1 -> L3-L4 LB Simscape/2, L3-L4 LB Moment/1

== system RBDmodel/L4-L5 AR readings ==
  L4-L5 AR Simscape Rotation : Inport
  L4-L5 AR Simscape Moment : Inport  Port=2
  L4-L5 AR Moment : Scope
  L4-L5 AR Rotation : Scope
  L4-L5 AR Simscape : Record  FileSettingsInternal="{\"entries\":[{\"content\":{\"excelSettings\":{\"content\":{},\"type\":\"Streamout.ExcelSettings\"}},\"type\":\"Streamout.FileSettingStorage\",\"uuid\":\"22ee5429-b0dc-4563-83b8-15fc97b18f1f\"}],\"packageUris\":[\"http://schema.mathworks.com/mf0/streamout_blocks/R2020a\"],\"version\":\"1.0\"}"  Layout=[1 1]  SignalsInternal="{\"entries\":[{\"content\":{\"signals\":[{\"content\":{\"blockPath\":[\"RBDmodel/L4-L5 AR readings/L4-L5 AR Simscape\"],\"dimensions\":[1],\"domain\":\"RBDmodel/L4-L5 AR readings/L4-L5 AR Simscape\",\"lineColor\":\"#a2142f\",\"port\":1,\"sid\":[\"\"],\"signalID\":1464,\"signalName\":\"L4-L5 AR Simscape Rotation\"},\"type\":\"RecordBlkView.Signal\",\"uuid\":\"878d9bd7-08b6-4dbd-bbe6-ed022d721c95\"},{\"content\":{\"blockPath\":[\"RBDmodel/L4-L5 AR readings/L4-L5 AR Simscape\"],\"dimensions\":[1],\"domain\":\"RBDmodel/L4-L5 AR readings/L4-L5 AR Simscape\",\"lineColor\":\"#139fff\",\"port\":2,\"sid\":[\"\"],\"signalID\":1468,\"signalName\":\"L4-L5 AR Simscape Moment\"},\"type\":\"RecordBlkView.Signal\",\"uuid\":\"8a0298d5-c88a-476b-907c-fa990a76708f\"}]},\"type\":\"RecordBlkView.InputSignals\",\"uuid\":\"d6c75fef-9b3d-4599-8e28-137f3ee6693b\"}],\"packageUris\":[\"http://schema.mathworks.com/mf0/streamout_blocks/R2020a\"],\"version\":\"1.0\"}"  VisualizationBindings="{\"xyplotplugin\":{\"info\":[{\"series\":[],\"subplotID\":1}]}}"  CompatibilityTag=XY
  wires:
  L4-L5 AR Simscape Moment/1 -> L4-L5 AR Simscape/2, L4-L5 AR Moment/1
  L4-L5 AR Simscape Rotation/1 -> L4-L5 AR Simscape/1, L4-L5 AR Rotation/1

== system RBDmodel/L4-L5 FE readings ==
  L4-L5 FE Simscape Rotation : Inport
  L4-L5 FE Simscape Moment : Inport  Port=2
  L4-L5 FE Moment : Scope
  L4-L5 FE Rotation : Scope
  L4-L5 FE Simscape : Record  FileSettingsInternal="{\"entries\":[{\"content\":{\"excelSettings\":{\"content\":{},\"type\":\"Streamout.ExcelSettings\"}},\"type\":\"Streamout.FileSettingStorage\",\"uuid\":\"f454a2f2-99ca-4f18-a30c-f3205bc0580a\"}],\"packageUris\":[\"http://schema.mathworks.com/mf0/streamout_blocks/R2020a\"],\"version\":\"1.0\"}"  Layout=[1 1]  SignalsInternal="{\"entries\":[{\"content\":{\"signals\":[{\"content\":{\"blockPath\":[\"RBDmodel/L4-L5 FE readings/L4-L5 FE Simscape\"],\"dimensions\":[1],\"domain\":\"RBDmodel/L4-L5 FE readings/L4-L5 FE Simscape\",\"lineColor\":\"#ff6929\",\"port\":1,\"sid\":[\"\"],\"signalID\":1472,\"signalName\":\"L4-L5 FE Simscape Rotation\"},\"type\":\"RecordBlkView.Signal\",\"uuid\":\"e8a0fb96-0d72-4bb5-8a74-2e1ca2d9ffc6\"},{\"content\":{\"blockPath\":[\"RBDmodel/L4-L5 FE readings/L4-L5 FE Simscape\"],\"dimensions\":[1],\"domain\":\"RBDmodel/L4-L5 FE readings/L4-L5 FE Simscape\",\"lineColor\":\"#b746ff\",\"port\":2,\"sid\":[\"\"],\"signalID\":1476,\"signalName\":\"L4-L5 FE Simscape Moment\"},\"type\":\"RecordBlkView.Signal\",\"uuid\":\"38f7bc10-c240-49b5-b10d-e818320bb029\"}]},\"type\":\"RecordBlkView.InputSignals\",\"uuid\":\"835f358a-1510-4530-8c68-112d53cbe8e6\"}],\"packageUris\":[\"http://schema.mathworks.com/mf0/streamout_blocks/R2020a\"],\"version\":\"1.0\"}"  VisualizationBindings="{\"xyplotplugin\":{\"info\":[{\"series\":[],\"subplotID\":1}]}}"  CompatibilityTag=XY
  wires:
  L4-L5 FE Simscape Rotation/1 -> L4-L5 FE Simscape/1, L4-L5 FE Rotation/1
  L4-L5 FE Simscape Moment/1 -> L4-L5 FE Simscape/2, L4-L5 FE Moment/1

== system RBDmodel/L4-L5 LB readings ==
  L4-L5 LB Simscape Rotation : Inport
  L4-L5 LB Simscape Moment : Inport  Port=2
  L4-L5 LB Moment : Scope
  L4-L5 LB Rotation : Scope
  L4-L5 LB Simscape : Record  FileSettingsInternal="{\"entries\":[{\"content\":{\"excelSettings\":{\"content\":{},\"type\":\"Streamout.ExcelSettings\"}},\"type\":\"Streamout.FileSettingStorage\",\"uuid\":\"bb960ea0-e781-41a9-8e2d-b5d562a32fcc\"}],\"packageUris\":[\"http://schema.mathworks.com/mf0/streamout_blocks/R2020a\"],\"version\":\"1.0\"}"  Layout=[1 1]  SignalsInternal="{\"entries\":[{\"content\":{\"signals\":[{\"content\":{\"blockPath\":[\"RBDmodel/L4-L5 LB readings/L4-L5 LB Simscape\"],\"dimensions\":[1],\"domain\":\"RBDmodel/L4-L5 LB readings/L4-L5 LB Simscape\",\"lineColor\":\"#64d413\",\"port\":1,\"sid\":[\"\"],\"signalID\":1480,\"signalName\":\"L4-L5 LB Simscape Rotation\"},\"type\":\"RecordBlkView.Signal\",\"uuid\":\"22de7d52-8035-411a-9a2b-f3b9142724f5\"},{\"content\":{\"blockPath\":[\"RBDmodel/L4-L5 LB readings/L4-L5 LB Simscape\"],\"dimensions\":[1],\"domain\":\"RBDmodel/L4-L5 LB readings/L4-L5 LB Simscape\",\"lineColor\":\"#ff13a6\",\"port\":2,\"sid\":[\"\"],\"signalID\":1484,\"signalName\":\"L4-L5 LB Simscape Moment\"},\"type\":\"RecordBlkView.Signal\",\"uuid\":\"383d6900-42c4-4fc6-b7d1-0d9889c8ab6e\"}]},\"type\":\"RecordBlkView.InputSignals\",\"uuid\":\"2938e1cf-c341-4359-a15a-45cb0798463a\"}],\"packageUris\":[\"http://schema.mathworks.com/mf0/streamout_blocks/R2020a\"],\"version\":\"1.0\"}"  VisualizationBindings="{\"xyplotplugin\":{\"info\":[{\"series\":[],\"subplotID\":1}]}}"  CompatibilityTag=XY
  wires:
  L4-L5 LB Simscape Moment/1 -> L4-L5 LB Simscape/2, L4-L5 LB Moment/1
  L4-L5 LB Simscape Rotation/1 -> L4-L5 LB Simscape/1, L4-L5 LB Rotation/1

== system RBDmodel/L5-S1 AR readings ==
  L5-S1 AR Simscape Rotation : Inport
  L5-S1 AR Simscape Moment : Inport  Port=2
  L5-S1 AR Moment : Scope
  L5-S1 AR Rotation : Scope
  L5-S1 AR Simscape : Record  FileSettingsInternal="{\"entries\":[{\"content\":{\"excelSettings\":{\"content\":{},\"type\":\"Streamout.ExcelSettings\"}},\"type\":\"Streamout.FileSettingStorage\",\"uuid\":\"0ea696ca-752a-4f49-aa19-aaf05f026397\"}],\"packageUris\":[\"http://schema.mathworks.com/mf0/streamout_blocks/R2020a\"],\"version\":\"1.0\"}"  Layout=[1 1]  SignalsInternal="{\"entries\":[{\"content\":{\"signals\":[{\"content\":{\"blockPath\":[\"RBDmodel/L5-S1 AR readings/L5-S1 AR Simscape\"],\"dimensions\":[1],\"domain\":\"RBDmodel/L5-S1 AR readings/L5-S1 AR Simscape\",\"lineColor\":\"#fe330a\",\"port\":1,\"sid\":[\"\"],\"signalID\":1488,\"signalName\":\"L5-S1 AR Simscape Rotation\"},\"type\":\"RecordBlkView.Signal\",\"uuid\":\"06c4b33e-9367-4592-8896-9c92fa525287\"},{\"content\":{\"blockPath\":[\"RBDmodel/L5-S1 AR readings/L5-S1 AR Simscape\"],\"dimensions\":[1],\"domain\":\"RBDmodel/L5-S1 AR readings/L5-S1 AR Simscape\",\"lineColor\":\"#22b573\",\"port\":2,\"sid\":[\"\"],\"signalID\":1492,\"signalName\":\"L5-S1 AR Simscape Moment\"},\"type\":\"RecordBlkView.Signal\",\"uuid\":\"d16694f8-f2f9-4028-9fff-3650000f65d0\"}]},\"type\":\"RecordBlkView.InputSignals\",\"uuid\":\"3143b92d-e313-43cf-bdf9-41690c51367a\"}],\"packageUris\":[\"http://schema.mathworks.com/mf0/streamout_blocks/R2020a\"],\"version\":\"1.0\"}"  VisualizationBindings="{\"xyplotplugin\":{\"info\":[{\"series\":[],\"subplotID\":1}]}}"  CompatibilityTag=XY
  wires:
  L5-S1 AR Simscape Rotation/1 -> L5-S1 AR Simscape/1, L5-S1 AR Rotation/1
  L5-S1 AR Simscape Moment/1 -> L5-S1 AR Simscape/2, L5-S1 AR Moment/1

== system RBDmodel/L5-S1 FE readings ==
  L5-S1 FE Simscape Rotation : Inport
  L5-S1 FE Simscape Moment : Inport  Port=2
  L5-S1 FE M-R : Record  FileSettingsInternal="{\"entries\":[{\"content\":{\"excelSettings\":{\"content\":{},\"type\":\"Streamout.ExcelSettings\"}},\"type\":\"Streamout.FileSettingStorage\",\"uuid\":\"03ebff2b-1b06-4da9-8d86-58934dddd7ed\"}],\"packageUris\":[\"http://schema.mathworks.com/mf0/streamout_blocks/R2020a\"],\"version\":\"1.0\"}"  Layout=[1 1]  SignalsInternal="{\"entries\":[{\"content\":{\"signals\":[{\"content\":{\"blockPath\":[\"RBDmodel/L5-S1 FE readings/L5-S1 FE M-R\"],\"dimensions\":[1],\"domain\":\"RBDmodel/L5-S1 FE readings/L5-S1 FE M-R\",\"lineColor\":\"#0072bd\",\"port\":1,\"sid\":[\"\"],\"signalID\":1496,\"signalName\":\"L5-S1 FE Simscape Rotation\"},\"type\":\"RecordBlkView.Signal\",\"uuid\":\"c7e72e11-37de-42ef-a9b7-f2962ab60bf4\"},{\"content\":{\"blockPath\":[\"RBDmodel/L5-S1 FE readings/L5-S1 FE M-R\"],\"dimensions\":[1],\"domain\":\"RBDmodel/L5-S1 FE readings/L5-S1 FE M-R\",\"lineColor\":\"#d95319\",\"port\":2,\"sid\":[\"\"],\"signalID\":1500,\"signalName\":\"L5-S1 FE Simscape Moment\"},\"type\":\"RecordBlkView.Signal\",\"uuid\":\"add62477-f2b6-486c-99c6-c8c2e70971f6\"}]},\"type\":\"RecordBlkView.InputSignals\",\"uuid\":\"6319f37a-fd76-41fb-b067-3cac434fc51d\"}],\"packageUris\":[\"http://schema.mathworks.com/mf0/streamout_blocks/R2020a\"],\"version\":\"1.0\"}"  VisualizationBindings="{\"xyplotplugin\":{\"info\":[{\"series\":[],\"subplotID\":1}]}}"  CompatibilityTag=XY
  L5-S1 FE Moment : Scope
  L5-S1 FE Rot : Scope
  wires:
  L5-S1 FE Simscape Rotation/1 -> L5-S1 FE M-R/1, L5-S1 FE Rot/1
  L5-S1 FE Simscape Moment/1 -> L5-S1 FE M-R/2, L5-S1 FE Moment/1

== system RBDmodel/L5-S1 LB readings ==
  L5-S1 LB Simscape Rotation : Inport
  L5-S1 LB Simscape Moment : Inport  Port=2
  L5-S1 LB Moment : Scope
  L5-S1 LB Rotation : Scope
  L5-S1 LB Simscape : Record  FileSettingsInternal="{\"entries\":[{\"content\":{\"excelSettings\":{\"content\":{},\"type\":\"Streamout.ExcelSettings\"}},\"type\":\"Streamout.FileSettingStorage\",\"uuid\":\"1fe1a201-205f-45ed-a2ea-47484a7c7520\"}],\"packageUris\":[\"http://schema.mathworks.com/mf0/streamout_blocks/R2020a\"],\"version\":\"1.0\"}"  Layout=[1 1]  SignalsInternal="{\"entries\":[{\"content\":{\"signals\":[{\"content\":{\"blockPath\":[\"RBDmodel/L5-S1 LB readings/L5-S1 LB Simscape\"],\"dimensions\":[1],\"domain\":\"RBDmodel/L5-S1 LB readings/L5-S1 LB Simscape\",\"lineColor\":\"#edb120\",\"port\":1,\"sid\":[\"\"],\"signalID\":1504,\"signalName\":\"L5-S1 LB Simscape Rotation\"},\"type\":\"RecordBlkView.Signal\",\"uuid\":\"49aeebf1-1927-4a21-994a-9ca18f7aa7fa\"},{\"content\":{\"blockPath\":[\"RBDmodel/L5-S1 LB readings/L5-S1 LB Simscape\"],\"dimensions\":[1],\"domain\":\"RBDmodel/L5-S1 LB readings/L5-S1 LB Simscape\",\"lineColor\":\"#7e2f8e\",\"port\":2,\"sid\":[\"\"],\"signalID\":1508,\"signalName\":\"L5-S1 LB Simscape Moment\"},\"type\":\"RecordBlkView.Signal\",\"uuid\":\"8bc219cc-eb50-434f-892d-b414add4c373\"}]},\"type\":\"RecordBlkView.InputSignals\",\"uuid\":\"ff8d54f0-9aa0-43f4-b435-da7ba4316801\"}],\"packageUris\":[\"http://schema.mathworks.com/mf0/streamout_blocks/R2020a\"],\"version\":\"1.0\"}"  VisualizationBindings="{\"xyplotplugin\":{\"info\":[{\"series\":[],\"subplotID\":1}]}}"  CompatibilityTag=XY
  wires:
  L5-S1 LB Simscape Moment/1 -> L5-S1 LB Simscape/2, L5-S1 LB Moment/1
  L5-S1 LB Simscape Rotation/1 -> L5-S1 LB Simscape/1, L5-S1 LB Rotation/1

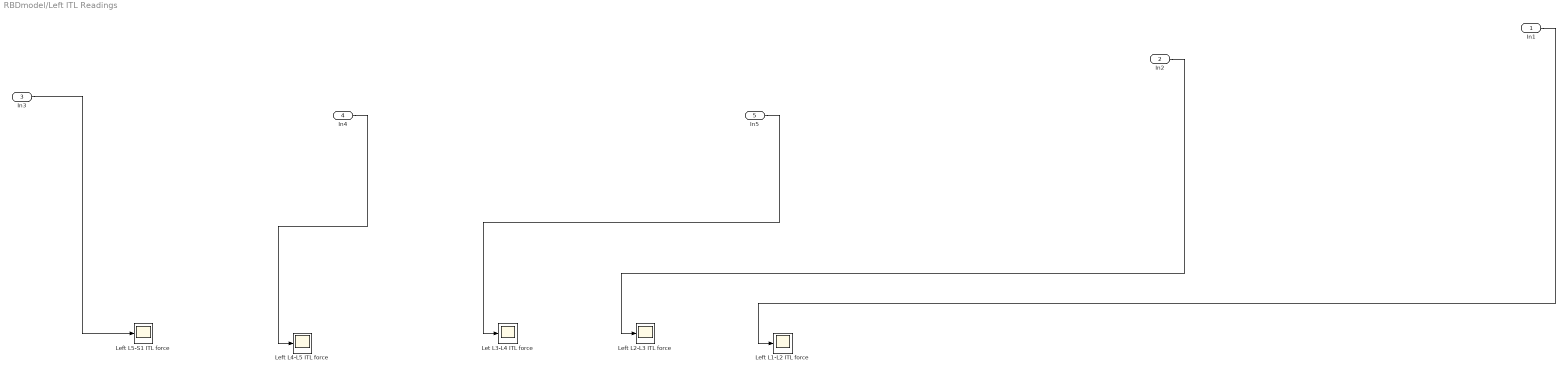
== system RBDmodel/Left ITL Readings ==
  In1 : Inport
  In2 : Inport  Port=2
  In3 : Inport  Port=3
  In4 : Inport  Port=4
  In5 : Inport  Port=5
  Left L1-L2 ITL force : Scope
  Left L2-L3 ITL force : Scope
  Left L4-L5 ITL force : Scope
  Left L5-S1 ITL force : Scope
  Let L3-L4 ITL force : Scope
  wires:
  In4/1 -> Left L4-L5 ITL force/1
  In1/1 -> Left L1-L2 ITL force/1
  In5/1 -> Let L3-L4 ITL force/1
  In3/1 -> Left L5-S1 ITL force/1
  In2/1 -> Left L2-L3 ITL force/1

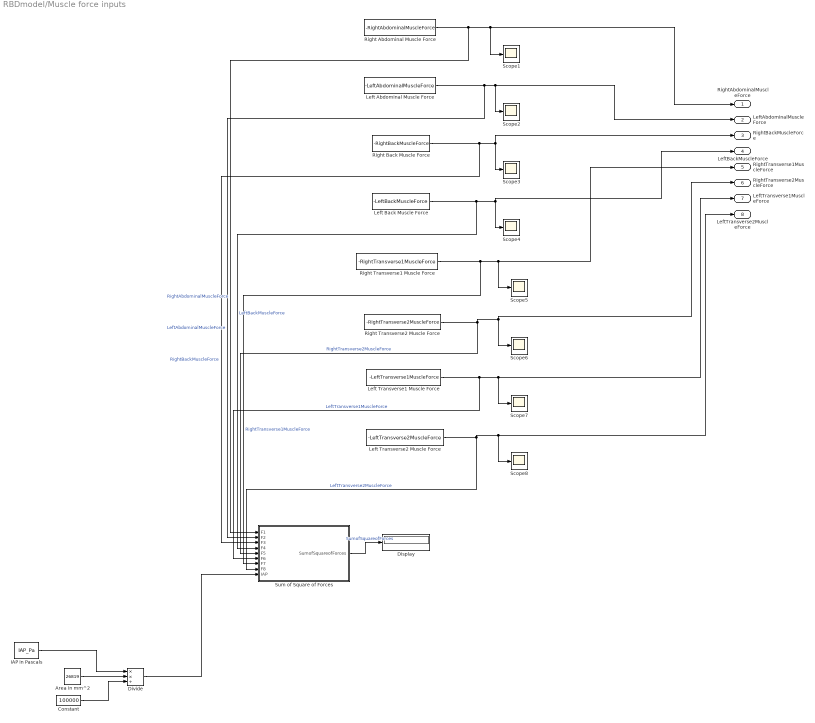
== system RBDmodel/Muscle force inputs ==
  Area in mm^2 : Constant  Value=26819
  Constant : Constant  Value=100000
  Display : Display
  Divide : Product  Inputs=**/
  IAP in Pascals : Constant  Value=IAP_Pa
  Left Abdominal Muscle Force : Constant  Value=-LeftAbdominalMuscleForce
  Left Back Muscle Force : Constant  Value=-LeftBackMuscleForce
  Left Transverse1 Muscle Force : Constant  Value=-LeftTransverse1MuscleForce
  Left Transverse2 Muscle Force : Constant  Value=-LeftTransverse2MuscleForce
  Right Abdominal Muscle Force : Constant  Value=-RightAbdominalMuscleForce
  Right Back Muscle Force : Constant  Value=-RightBackMuscleForce
  Right Transverse1 Muscle Force : Constant  Value=-RightTransverse1MuscleForce
  Right Transverse2 Muscle Force : Constant  Value=-RightTransverse2MuscleForce
  Scope{1..8} (8 alike) : Scope
  Sum of Square of Forces : MATLAB Function  TreatAsAtomicUnit=on
  RightAbdominalMuscleForce : Outport
  LeftAbdominalMuscleForce : Outport  Port=2
  RightBackMuscleForce : Outport  Port=3
  LeftBackMuscleForce : Outport  Port=4
  RightTransverse1MuscleForce : Outport  Port=5
  RightTransverse2MuscleForce : Outport  Port=6
  LeftTransverse1MuscleForce : Outport  Port=7
  LeftTransverse2MuscleForce : Outport  Port=8
  wires:
  Left Transverse2 Muscle Force/1 -> LeftTransverse2MuscleForce/1, Scope8/1, Sum of Square of Forces/8(F8)  "LeftTransverse2MuscleForce"
  Left Abdominal Muscle Force/1 -> LeftAbdominalMuscleForce/1, Scope2/1, Sum of Square of Forces/2(F2)  "LeftAbdominalMuscleForce"
  Sum of Square of Forces/1(SumofSquareofForces) -> Display/1  "SumofSquareofForces"
  Area in mm^2/1 -> Divide/2
  Left Back Muscle Force/1 -> Sum of Square of Forces/4(F4), LeftBackMuscleForce/1, Scope4/1  "LeftBackMuscleForce"
  Divide/1 -> Sum of Square of Forces/9(IAP)
  Left Transverse1 Muscle Force/1 -> LeftTransverse1MuscleForce/1, Scope7/1, Sum of Square of Forces/6(F6)  "LeftTransverse1MuscleForce"
  Right Abdominal Muscle Force/1 -> RightAbdominalMuscleForce/1, Scope1/1, Sum of Square of Forces/1(F1)  "RightAbdominalMuscleForce"
  Right Back Muscle Force/1 -> RightBackMuscleForce/1, Scope3/1, Sum of Square of Forces/3(F3)  "RightBackMuscleForce"
  Right Transverse2 Muscle Force/1 -> RightTransverse2MuscleForce/1, Scope6/1, Sum of Square of Forces/5(F5)  "RightTransverse2MuscleForce"
  Right Transverse1 Muscle Force/1 -> RightTransverse1MuscleForce/1, Scope5/1, Sum of Square of Forces/7(F7)  "RightTransverse1MuscleForce"
  IAP in Pascals/1 -> Divide/1
  Constant/1 -> Divide/3

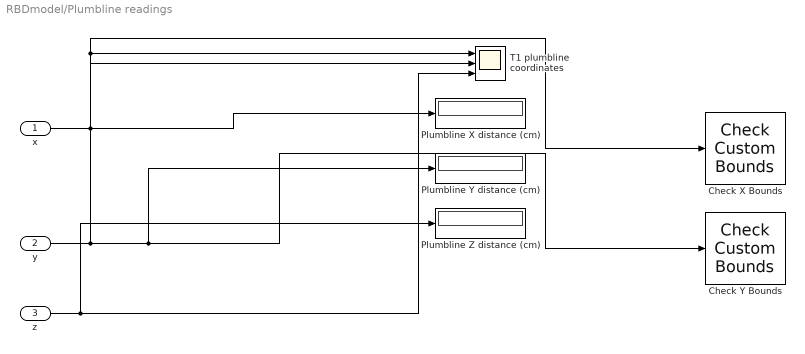
== system RBDmodel/Plumbline readings ==
  x : Inport
  y : Inport  Port=2
  z : Inport  Port=3
  Check X Bounds : checkpacklib/Check Custom Bounds  InstantiateOnLoad=on  enabled=off  stopWhenAssertionFail=off  export=off  ViewDlgPos=[983.4 172.2 510.4 379.2]  OpenViewOnLoad=off  LaunchViewOnOpen=off  TimeUnits=seconds  EnableUpperBound=on  UpperBoundTimes=[0 3]  UpperBoundAmplitudes=[2 2];  EnableLowerBound=on  LowerBoundTimes=[0 3]  LowerBoundAmplitudes=[-2 -2]
      settings: LibrarySourceBlock=sdolib/Signal Constraints/Check Custom Bounds
  Check Y Bounds : checkpacklib/Check Custom Bounds  InstantiateOnLoad=on  enabled=off  stopWhenAssertionFail=off  export=off  ViewDlgPos=[509 222 510 390]  OpenViewOnLoad=off  LaunchViewOnOpen=off  TimeUnits=seconds  EnableUpperBound=on  UpperBoundTimes=[0 3]  UpperBoundAmplitudes=[2 2];  EnableLowerBound=on  LowerBoundTimes=[0 3]  LowerBoundAmplitudes=[-2 -2]
      settings: LibrarySourceBlock=sdolib/Signal Constraints/Check Custom Bounds
  Plumbline X distance (cm) : Display
  Plumbline Y distance (cm) : Display
  Plumbline Z distance (cm) : Display
  T1 plumbline coordinates : Scope  NumInputPorts=3
  wires:
  x/1 -> Plumbline X distance (cm)/1, Check X Bounds/1, T1 plumbline coordinates/1
  z/1 -> Plumbline Z distance (cm)/1, T1 plumbline coordinates/3
  y/1 -> Plumbline Y distance (cm)/1, Check Y Bounds/1, T1 plumbline coordinates/2

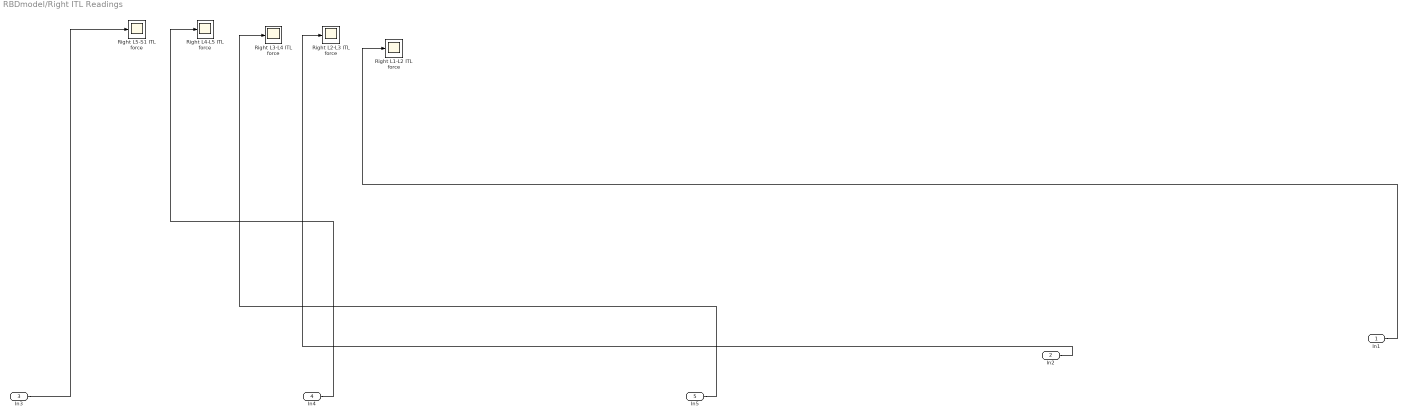
== system RBDmodel/Right ITL Readings ==
  In1 : Inport
  In2 : Inport  Port=2
  In3 : Inport  Port=3
  In4 : Inport  Port=4
  In5 : Inport  Port=5
  Right L1-L2 ITL force : Scope
  Right L2-L3 ITL force : Scope
  Right L3-L4 ITL force : Scope
  Right L4-L5 ITL force : Scope
  Right L5-S1 ITL force : Scope
  wires:
  In5/1 -> Right L3-L4 ITL force/1
  In3/1 -> Right L5-S1 ITL force/1
  In2/1 -> Right L2-L3 ITL force/1
  In1/1 -> Right L1-L2 ITL force/1
  In4/1 -> Right L4-L5 ITL force/1

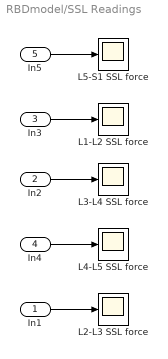
== system RBDmodel/SSL Readings ==
  In1 : Inport
  In2 : Inport  Port=2
  In3 : Inport  Port=3
  In4 : Inport  Port=4
  In5 : Inport  Port=5
  L1-L2 SSL force : Scope
  L2-L3 SSL force : Scope
  L3-L4 SSL force : Scope
  L4-L5 SSL force : Scope
  L5-S1 SSL force : Scope
  wires:
  In5/1 -> L5-S1 SSL force/1
  In3/1 -> L1-L2 SSL force/1
  In1/1 -> L2-L3 SSL force/1
  In2/1 -> L3-L4 SSL force/1
  In4/1 -> L4-L5 SSL force/1
